simulink model "lab3_car1"  (R2022b)
settings: Solver=VariableStepAuto  StartTime=0.0  StopTime=30.0  RelTol=1e-3
settings Model: Creator=mluser  LastModifiedBy=mluser

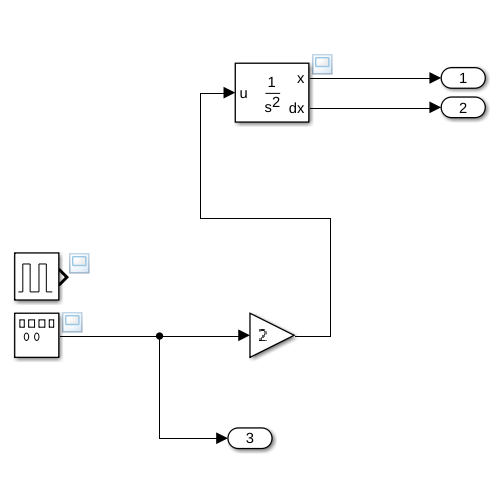
[thumbnail: Simulink's stored preview of the top-level diagram]
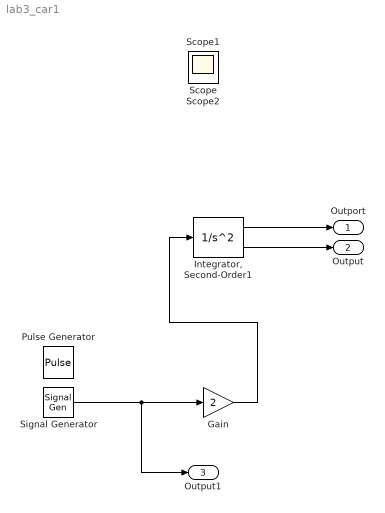
== system lab3_car1 ==
  Gain : Gain  Gain=2
  "Integrator, Second-Order1" : SecondOrderIntegrator
  Pulse Generator : DiscretePulseGenerator  PulseType=Time based  Period=10  PulseWidth=5
  Signal Generator : SignalGenerator  WaveForm=square  Units=rad/sec
  Outport : Outport
  Output : Outport  Port=2
  Output1 : Outport  Port=3
  Scope : Scope
  Scope1 : Scope
  Scope2 : Scope
  wires:
  Signal Generator/1 -> Gain/1, Output1/1
  Gain/1 -> "Integrator, Second-Order1"/1
  "Integrator, Second-Order1"/2 -> Output/1
  "Integrator, Second-Order1"/1 -> Outport/1
